simulink model "control_mimo_simulink"  (R2019b)
settings: Solver=ode45  StartTime=0.0  StopTime=60  MaxStep=0.001  RelTol=1e-3
values from neighbouring files (symbols this model uses):
  A = jacobian(F,X)    [codigo_pto_equilibrio_no_lineal.m]
  AL = sys.a    [codigo_pto_equilibrio_no_lineal.m]
  B = jacobian(F,U)    [codigo_pto_equilibrio_no_lineal.m]
  BL = double(Bp)    [codigo_pto_equilibrio_no_lineal.m]
  CL = [2 1 0 ... (first row only)    [codigo_pto_equilibrio_no_lineal.m]
  DL = [0 0 0 ... (first row only)    [codigo_pto_equilibrio_no_lineal.m]
  Kest = Grand*inv(X)    [codigo_pto_equilibrio_no_lineal.m]
  u10 = 1    [codigo_pto_equilibrio_no_lineal.m]
  u20 = 2    [codigo_pto_equilibrio_no_lineal.m]
  u30 = 3    [codigo_pto_equilibrio_no_lineal.m]
  x10n = sqrt((x20n+u20*u30)/a)    [codigo_pto_equilibrio_no_lineal.m]
  x20n = b*x30n - u10*u30    [codigo_pto_equilibrio_no_lineal.m]
  x30n = sqrt((exp(-u10))/c)    [codigo_pto_equilibrio_no_lineal.m]
  xini = [0.2; 0.3; 0.01]    [codigo_pto_equilibrio_no_lineal.m]
undefined symbols (not defined in the file or in its folder): C, D, Kes, Ki
libraries: cstblocks x26
settings Model: Creator=B13  LastModifiedBy=KEVIN ALEJANDRO

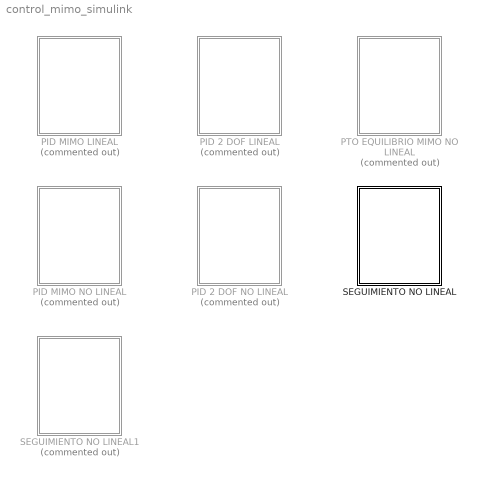
== system control_mimo_simulink ==
  PID 2 DOF LINEAL : Subsystem  Commented=on
  PID 2 DOF NO LINEAL : Subsystem  Commented=on
  PID MIMO LINEAL : Subsystem  Commented=on
  PID MIMO NO LINEAL : Subsystem  Commented=on
  PTO EQUILIBRIO MIMO NO LINEAL : Subsystem  Commented=on
  SEGUIMIENTO NO LINEAL : Subsystem
  SEGUIMIENTO NO LINEAL1 : Subsystem  Commented=on

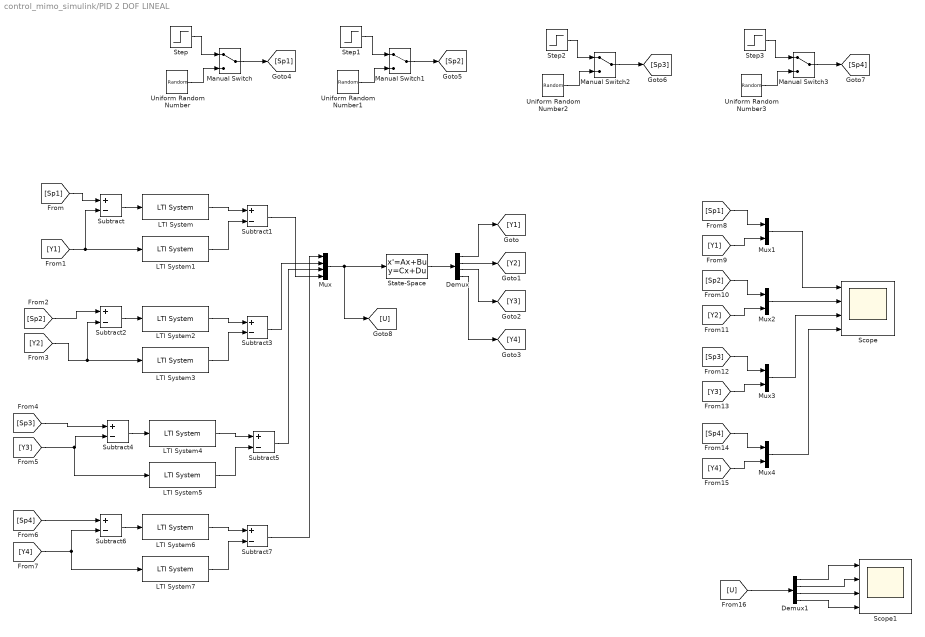
== system control_mimo_simulink/PID 2 DOF LINEAL ==
  Demux : Demux
  Demux1 : Demux
  LTI System : cstblocks/LTI System  sys=C14a  IC=[]
  LTI System1 : cstblocks/LTI System  sys=C14b  IC=[]
  LTI System2 : cstblocks/LTI System  sys=C22a  IC=[]
  LTI System3 : cstblocks/LTI System  sys=C22b  IC=[]
  LTI System4 : cstblocks/LTI System  sys=C33a  IC=[]
  LTI System5 : cstblocks/LTI System  sys=C33b  IC=[]
  LTI System6 : cstblocks/LTI System  sys=C41a  IC=[]
  LTI System7 : cstblocks/LTI System  sys=C41b  IC=[]
  Manual Switch{,1..3} (4 alike) : ManualSwitch
  Mux : Mux
  Mux{1..4} (4 alike) : Mux  Inputs=2
  Scope : Scope  NumInputPorts=4
  Scope1 : Scope  NumInputPorts=4
  State-Space : StateSpace  A=A  B=B  C=C  D=D  InitialCondition=xini
  Step{,1..3} (4 alike) : Step  Time=0  After=0  SampleTime=0
  Subtract{,1..7} (8 alike) : Sum  Inputs=+-
  Uniform Random Number : UniformRandomNumber  SampleTime=500
  Uniform Random Number1 : UniformRandomNumber  SampleTime=700
  Uniform Random Number2 : UniformRandomNumber  SampleTime=900
  Uniform Random Number3 : UniformRandomNumber  SampleTime=1100
  wires:
  Mux2/1 -> Scope/2
  Step1/1 -> Manual Switch1/1
  Manual Switch/1 -> [Sp1]
  [U] -> Demux1/1
  Step2/1 -> Manual Switch2/1
  [Sp2] -> Mux2/1
  Uniform Random Number/1 -> Manual Switch/2
  [Y3] -> Mux3/2
  Demux/4 -> [Y4]
  Mux/1 -> [U], State-Space/1
  Step3/1 -> Manual Switch3/1
  Manual Switch2/1 -> [Sp3]
  Manual Switch1/1 -> [Sp2]
  Manual Switch3/1 -> [Sp4]
  Mux3/1 -> Scope/3
  Uniform Random Number2/1 -> Manual Switch2/2
  Uniform Random Number3/1 -> Manual Switch3/2
  Uniform Random Number1/1 -> Manual Switch1/2
  Step/1 -> Manual Switch/1
  Demux/2 -> [Y2]
  [Y4] -> Mux4/2
  [Sp1] -> Mux1/1
  [Sp4] -> Mux4/1
  Demux/3 -> [Y3]
  State-Space/1 -> Demux/1
  Demux/1 -> [Y1]
  Demux1/3 -> Scope1/3
  Demux1/1 -> Scope1/1
  Demux1/4 -> Scope1/4
  [Sp3] -> Mux3/1
  [Y1] -> Mux1/2
  Mux1/1 -> Scope/1
  Mux4/1 -> Scope/4
  [Y2] -> Mux2/2
  Demux1/2 -> Scope1/2
  [Sp1] -> Subtract/1
  [Y1] -> Subtract/2, LTI System1/1
  Subtract/1 -> LTI System/1
  LTI System/1 -> Subtract1/1
  LTI System1/1 -> Subtract1/2
  Subtract1/1 -> Mux/4
  [Y2] -> Subtract2/2, LTI System3/1
  [Sp2] -> Subtract2/1
  LTI System3/1 -> Subtract3/2
  LTI System2/1 -> Subtract3/1
  Subtract2/1 -> LTI System2/1
  Subtract3/1 -> Mux/2
  [Sp3] -> Subtract4/1
  LTI System5/1 -> Subtract5/2
  LTI System4/1 -> Subtract5/1
  Subtract4/1 -> LTI System4/1
  [Y3] -> LTI System5/1, Subtract4/2
  Subtract5/1 -> Mux/3
  [Sp4] -> Subtract6/1
  LTI System7/1 -> Subtract7/2
  LTI System6/1 -> Subtract7/1
  Subtract6/1 -> LTI System6/1
  [Y4] -> Subtract6/2, LTI System7/1
  Subtract7/1 -> Mux/1

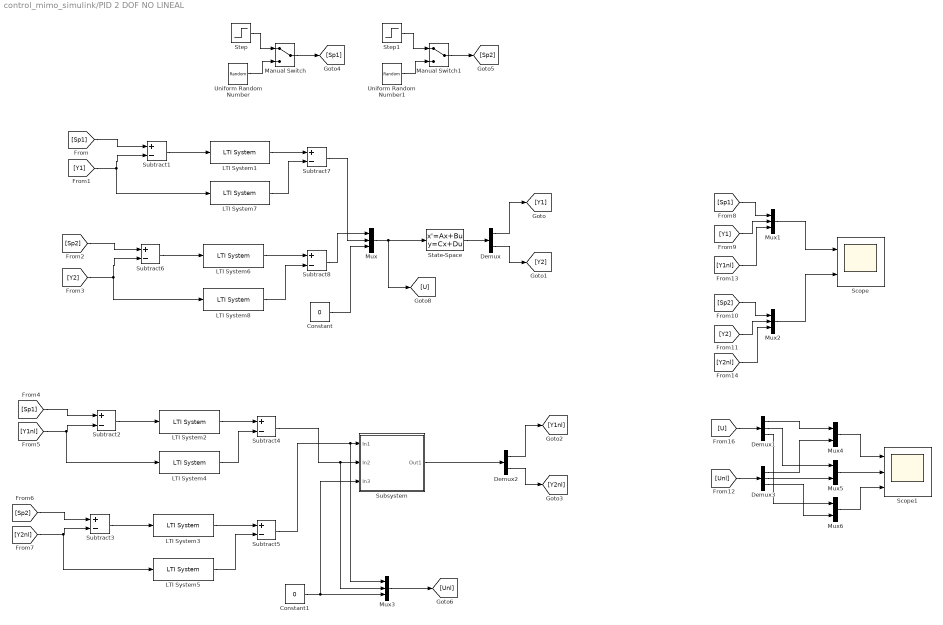
== system control_mimo_simulink/PID 2 DOF NO LINEAL ==
  Constant : Constant  Value=0
  Constant1 : Constant  Value=0
  Demux : Demux  Outputs=2
  Demux1 : Demux  Outputs=3
  Demux2 : Demux  Outputs=2
  Demux3 : Demux  Outputs=3
  LTI System1 : cstblocks/LTI System  sys=C12a  IC=[]
  LTI System2 : cstblocks/LTI System  sys=C12a  IC=[]
  LTI System3 : cstblocks/LTI System  sys=C21a  IC=[]
  LTI System4 : cstblocks/LTI System  sys=C12b  IC=[]
  LTI System5 : cstblocks/LTI System  sys=C21b  IC=[]
  LTI System6 : cstblocks/LTI System  sys=C21a  IC=[]
  LTI System7 : cstblocks/LTI System  sys=C12b  IC=[]
  LTI System8 : cstblocks/LTI System  sys=C21b  IC=[]
  Manual Switch : ManualSwitch
  Manual Switch1 : ManualSwitch
  Mux{,1..3} (4 alike) : Mux  Inputs=3
  Mux4 : Mux  Inputs=2
  Mux5 : Mux  Inputs=2
  Mux6 : Mux  Inputs=2
  Scope : Scope  NumInputPorts=2
  Scope1 : Scope  NumInputPorts=3
  State-Space : StateSpace  A=AL  B=BL  C=CL  D=DL  InitialCondition=xini
  Step : Step  Time=0  After=0  SampleTime=0
  Step1 : Step  Time=0  After=0  SampleTime=0
  Subsystem : Subsystem
  Subtract{1..8} (8 alike) : Sum  Inputs=+-
  Uniform Random Number : UniformRandomNumber  Minimum=-10  Maximum=10  SampleTime=5
  Uniform Random Number1 : UniformRandomNumber  Minimum=-10  Maximum=10  SampleTime=8
  wires:
  Mux2/1 -> Scope/2
  Step1/1 -> Manual Switch1/1
  Manual Switch/1 -> [Sp1]
  [U] -> Demux1/1
  [Sp2] -> Mux2/1
  Uniform Random Number/1 -> Manual Switch/2
  Mux/1 -> [U], State-Space/1
  Manual Switch1/1 -> [Sp2]
  Uniform Random Number1/1 -> Manual Switch1/2
  Step/1 -> Manual Switch/1
  Demux/2 -> [Y2]
  [Sp1] -> Mux1/1
  State-Space/1 -> Demux/1
  Demux/1 -> [Y1]
  [Y1] -> Mux1/2
  Mux1/1 -> Scope/1
  [Y2] -> Mux2/2
  Constant/1 -> Mux/3
  Subtract3/1 -> LTI System3/1
  Demux2/2 -> [Y2nl]
  [Sp1] -> Subtract2/1
  [Y1nl] -> LTI System4/1, Subtract2/2
  Subtract2/1 -> LTI System2/1
  [Sp2] -> Subtract3/1
  Subsystem/1(Out1) -> Demux2/1
  Demux2/1 -> [Y1nl]
  Mux3/1 -> [Unl]
  [Y2nl] -> LTI System5/1, Subtract3/2
  Constant1/1 -> Subsystem/3(In3), Mux3/3
  [Unl] -> Demux3/1
  Demux1/1 -> Mux4/1
  Demux3/1 -> Mux4/2
  Demux1/2 -> Mux5/1
  Demux3/2 -> Mux5/2
  Demux1/3 -> Mux6/1
  Demux3/3 -> Mux6/2
  Mux5/1 -> Scope1/2
  Mux4/1 -> Scope1/1
  Mux6/1 -> Scope1/3
  [Y1nl] -> Mux1/3
  [Y2nl] -> Mux2/3
  LTI System2/1 -> Subtract4/1
  LTI System4/1 -> Subtract4/2
  Subtract4/1 -> Mux3/2, Subsystem/2(In2)
  LTI System3/1 -> Subtract5/1
  LTI System5/1 -> Subtract5/2
  Subtract5/1 -> Mux3/1, Subsystem/1(In1)
  [Y1] -> Subtract1/2, LTI System7/1
  LTI System7/1 -> Subtract7/2
  LTI System8/1 -> Subtract8/2
  Subtract6/1 -> LTI System6/1
  [Sp2] -> Subtract6/1
  LTI System1/1 -> Subtract7/1
  [Sp1] -> Subtract1/1
  LTI System6/1 -> Subtract8/1
  [Y2] -> Subtract6/2, LTI System8/1
  Subtract1/1 -> LTI System1/1
  Subtract7/1 -> Mux/2
  Subtract8/1 -> Mux/1

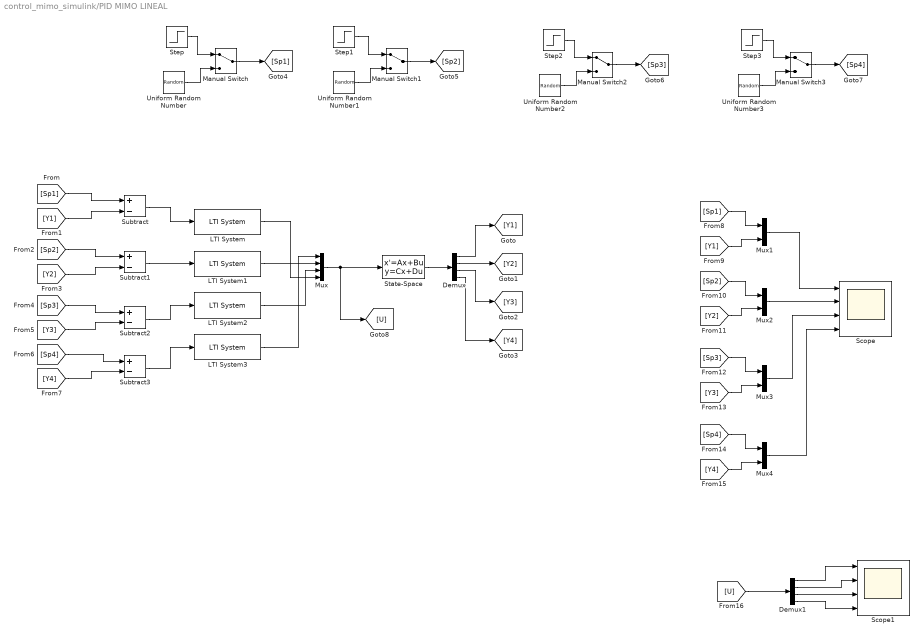
== system control_mimo_simulink/PID MIMO LINEAL ==
  Demux : Demux
  Demux1 : Demux
  LTI System : cstblocks/LTI System  sys=C14  IC=[]
  LTI System1 : cstblocks/LTI System  sys=C22  IC=[]
  LTI System2 : cstblocks/LTI System  sys=C33  IC=[]
  LTI System3 : cstblocks/LTI System  sys=C41  IC=[]
  Manual Switch{,1..3} (4 alike) : ManualSwitch
  Mux : Mux
  Mux{1..4} (4 alike) : Mux  Inputs=2
  Scope : Scope  NumInputPorts=4
  Scope1 : Scope  NumInputPorts=4
  State-Space : StateSpace  A=A  B=B  C=C  D=D  InitialCondition=xini
  Step{,1..3} (4 alike) : Step  Time=0  After=0  SampleTime=0
  Subtract{,1..3} (4 alike) : Sum  Inputs=+-
  Uniform Random Number : UniformRandomNumber  SampleTime=500
  Uniform Random Number1 : UniformRandomNumber  SampleTime=700
  Uniform Random Number2 : UniformRandomNumber  SampleTime=900
  Uniform Random Number3 : UniformRandomNumber  SampleTime=1100
  wires:
  Mux2/1 -> Scope/2
  Step1/1 -> Manual Switch1/1
  Manual Switch/1 -> [Sp1]
  [Y1] -> Subtract/2
  [U] -> Demux1/1
  LTI System/1 -> Mux/4
  Step2/1 -> Manual Switch2/1
  [Sp2] -> Mux2/1
  Uniform Random Number/1 -> Manual Switch/2
  [Y3] -> Mux3/2
  Demux/4 -> [Y4]
  Mux/1 -> [U], State-Space/1
  Step3/1 -> Manual Switch3/1
  Subtract2/1 -> LTI System2/1
  LTI System1/1 -> Mux/2
  Manual Switch2/1 -> [Sp3]
  Manual Switch1/1 -> [Sp2]
  Subtract3/1 -> LTI System3/1
  Manual Switch3/1 -> [Sp4]
  Mux3/1 -> Scope/3
  Subtract1/1 -> LTI System1/1
  Uniform Random Number2/1 -> Manual Switch2/2
  Uniform Random Number3/1 -> Manual Switch3/2
  Uniform Random Number1/1 -> Manual Switch1/2
  Step/1 -> Manual Switch/1
  [Y3] -> Subtract2/2
  [Sp1] -> Subtract/1
  Demux/2 -> [Y2]
  [Y4] -> Mux4/2
  [Sp1] -> Mux1/1
  LTI System2/1 -> Mux/3
  [Sp4] -> Mux4/1
  [Y2] -> Subtract1/2
  [Sp2] -> Subtract1/1
  Demux/3 -> [Y3]
  [Sp3] -> Subtract2/1
  Subtract/1 -> LTI System/1
  [Sp4] -> Subtract3/1
  State-Space/1 -> Demux/1
  LTI System3/1 -> Mux/1
  [Y4] -> Subtract3/2
  Demux/1 -> [Y1]
  Demux1/3 -> Scope1/3
  Demux1/1 -> Scope1/1
  Demux1/4 -> Scope1/4
  [Sp3] -> Mux3/1
  [Y1] -> Mux1/2
  Mux1/1 -> Scope/1
  Mux4/1 -> Scope/4
  [Y2] -> Mux2/2
  Demux1/2 -> Scope1/2

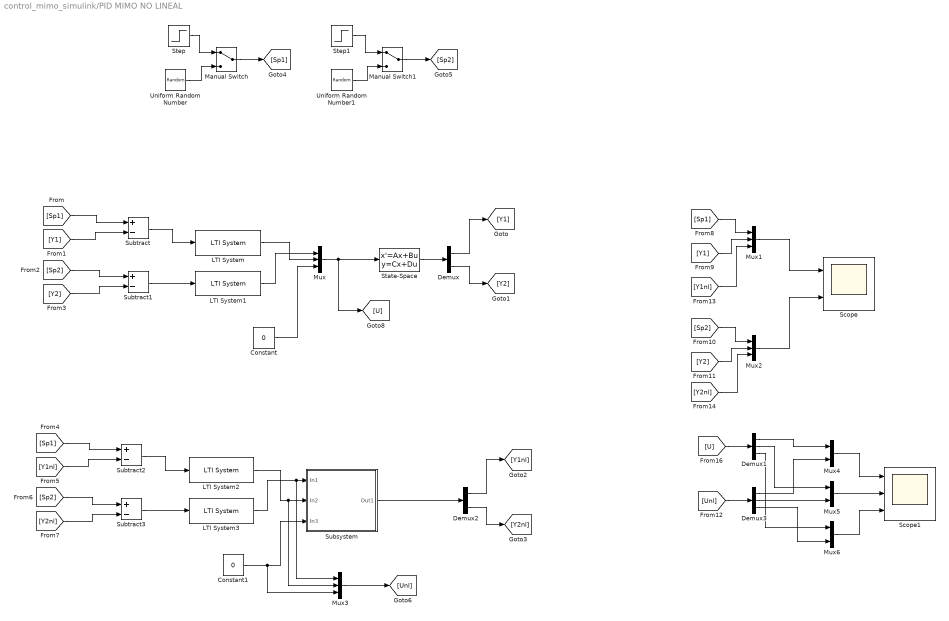
== system control_mimo_simulink/PID MIMO NO LINEAL ==
  Constant : Constant  Value=0
  Constant1 : Constant  Value=0
  Demux : Demux  Outputs=2
  Demux1 : Demux  Outputs=3
  Demux2 : Demux  Outputs=2
  Demux3 : Demux  Outputs=3
  LTI System : cstblocks/LTI System  sys=C12  IC=[]
  LTI System1 : cstblocks/LTI System  sys=C21  IC=[]
  LTI System2 : cstblocks/LTI System  sys=C12  IC=[]
  LTI System3 : cstblocks/LTI System  sys=C21  IC=[]
  Manual Switch : ManualSwitch
  Manual Switch1 : ManualSwitch
  Mux{,1..3} (4 alike) : Mux  Inputs=3
  Mux4 : Mux  Inputs=2
  Mux5 : Mux  Inputs=2
  Mux6 : Mux  Inputs=2
  Scope : Scope  NumInputPorts=2
  Scope1 : Scope  NumInputPorts=3
  State-Space : StateSpace  A=AL  B=BL  C=CL  D=DL  InitialCondition=xini
  Step : Step  Time=0  After=0  SampleTime=0
  Step1 : Step  Time=0  After=0  SampleTime=0
  Subsystem : Subsystem
  Subtract{,1..3} (4 alike) : Sum  Inputs=+-
  Uniform Random Number : UniformRandomNumber  Minimum=-2  Maximum=2  SampleTime=5
  Uniform Random Number1 : UniformRandomNumber  Minimum=-2  Maximum=2  SampleTime=8
  wires:
  Mux2/1 -> Scope/2
  Step1/1 -> Manual Switch1/1
  Manual Switch/1 -> [Sp1]
  [Y1] -> Subtract/2
  [U] -> Demux1/1
  [Sp2] -> Mux2/1
  Uniform Random Number/1 -> Manual Switch/2
  Mux/1 -> [U], State-Space/1
  Manual Switch1/1 -> [Sp2]
  Subtract1/1 -> LTI System1/1
  Uniform Random Number1/1 -> Manual Switch1/2
  Step/1 -> Manual Switch/1
  [Sp1] -> Subtract/1
  Demux/2 -> [Y2]
  [Sp1] -> Mux1/1
  [Y2] -> Subtract1/2
  [Sp2] -> Subtract1/1
  Subtract/1 -> LTI System/1
  State-Space/1 -> Demux/1
  Demux/1 -> [Y1]
  [Y1] -> Mux1/2
  Mux1/1 -> Scope/1
  [Y2] -> Mux2/2
  LTI System/1 -> Mux/2
  LTI System1/1 -> Mux/1
  Constant/1 -> Mux/3
  Subtract3/1 -> LTI System3/1
  Demux2/2 -> [Y2nl]
  [Sp1] -> Subtract2/1
  [Y1nl] -> Subtract2/2
  Subtract2/1 -> LTI System2/1
  [Sp2] -> Subtract3/1
  Subsystem/1(Out1) -> Demux2/1
  Demux2/1 -> [Y1nl]
  Mux3/1 -> [Unl]
  [Y2nl] -> Subtract3/2
  LTI System2/1 -> Mux3/2, Subsystem/2(In2)
  LTI System3/1 -> Mux3/1, Subsystem/1(In1)
  Constant1/1 -> Mux3/3, Subsystem/3(In3)
  [Unl] -> Demux3/1
  Demux1/1 -> Mux4/1
  Demux3/1 -> Mux4/2
  Demux1/2 -> Mux5/1
  Demux3/2 -> Mux5/2
  Demux1/3 -> Mux6/1
  Demux3/3 -> Mux6/2
  Mux5/1 -> Scope1/2
  Mux4/1 -> Scope1/1
  Mux6/1 -> Scope1/3
  [Y1nl] -> Mux1/3
  [Y2nl] -> Mux2/3

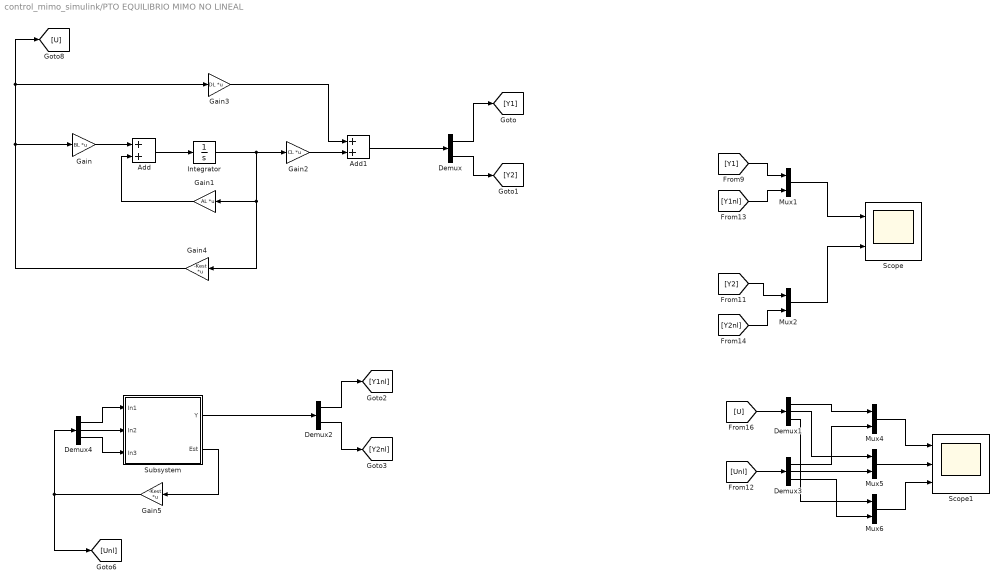
== system control_mimo_simulink/PTO EQUILIBRIO MIMO NO LINEAL ==
  Add : Sum
  Add1 : Sum
  Demux : Demux  Outputs=2
  Demux1 : Demux  Outputs=3
  Demux2 : Demux  Outputs=2
  Demux3 : Demux  Outputs=3
  Demux4 : Demux  Outputs=3
  Gain : Gain  Gain=BL  Multiplication=Matrix(K*u)
  Gain1 : Gain  Gain=AL  Multiplication=Matrix(K*u)
  Gain2 : Gain  Gain=CL  Multiplication=Matrix(K*u)
  Gain3 : Gain  Gain=DL  Multiplication=Matrix(K*u)
  Gain4 : Gain  Gain=-Kest  Multiplication=Matrix(K*u)
  Gain5 : Gain  Gain=-Kest  Multiplication=Matrix(K*u)
  Integrator : Integrator  InitialCondition=xini
  Mux{1..2,4..6} (5 alike) : Mux  Inputs=2
  Scope : Scope  NumInputPorts=2
  Scope1 : Scope  NumInputPorts=3
  Subsystem : Subsystem
  wires:
  Mux2/1 -> Scope/2
  [U] -> Demux1/1
  Demux/2 -> [Y2]
  Add1/1 -> Demux/1
  Demux/1 -> [Y1]
  Mux1/1 -> Scope/1
  Demux2/2 -> [Y2nl]
  Subsystem/1(Y) -> Demux2/1
  Demux2/1 -> [Y1nl]
  [Unl] -> Demux3/1
  Demux1/1 -> Mux4/1
  Demux3/1 -> Mux4/2
  Demux1/2 -> Mux5/1
  Demux3/2 -> Mux5/2
  Demux1/3 -> Mux6/1
  Demux3/3 -> Mux6/2
  Mux5/1 -> Scope1/2
  Mux4/1 -> Scope1/1
  Mux6/1 -> Scope1/3
  Gain/1 -> Add/1
  Add/1 -> Integrator/1
  Gain1/1 -> Add/2
  Integrator/1 -> Gain2/1, Gain4/1, Gain1/1
  Gain2/1 -> Add1/2
  Gain3/1 -> Add1/1
  Gain4/1 -> Gain/1, [U], Gain3/1
  Subsystem/2(Est) -> Gain5/1
  Demux4/2 -> Subsystem/2(In2)
  Demux4/1 -> Subsystem/1(In1)
  Demux4/3 -> Subsystem/3(In3)
  Gain5/1 -> Demux4/1, [Unl]
  [Y1] -> Mux1/1
  [Y1nl] -> Mux1/2
  [Y2] -> Mux2/1
  [Y2nl] -> Mux2/2

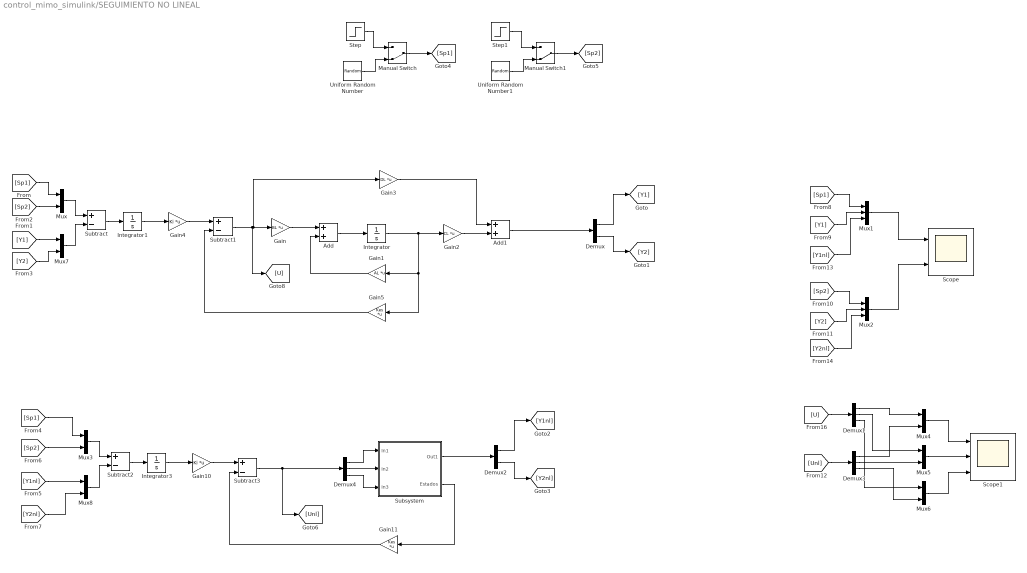
== system control_mimo_simulink/SEGUIMIENTO NO LINEAL ==
  Add : Sum
  Add1 : Sum
  Demux : Demux  Outputs=2
  Demux1 : Demux  Outputs=3
  Demux2 : Demux  Outputs=2
  Demux3 : Demux  Outputs=3
  Demux4 : Demux  Outputs=3
  Gain : Gain  Gain=BL  Multiplication=Matrix(K*u)
  Gain1 : Gain  Gain=AL  Multiplication=Matrix(K*u)
  Gain10 : Gain  Gain=Ki  Multiplication=Matrix(K*u)
  Gain11 : Gain  Gain=Kes  Multiplication=Matrix(K*u)
  Gain2 : Gain  Gain=CL  Multiplication=Matrix(K*u)
  Gain3 : Gain  Gain=DL  Multiplication=Matrix(K*u)
  Gain4 : Gain  Gain=Ki  Multiplication=Matrix(K*u)
  Gain5 : Gain  Gain=Kes  Multiplication=Matrix(K*u)
  Integrator : Integrator
  Integrator1 : Integrator
  Integrator3 : Integrator
  Manual Switch : ManualSwitch  CurrentSetting=0
  Manual Switch1 : ManualSwitch  CurrentSetting=0
  Mux{,3..8} (7 alike) : Mux  Inputs=2
  Mux1 : Mux  Inputs=3
  Mux2 : Mux  Inputs=3
  Scope : Scope  NumInputPorts=2
  Scope1 : Scope  NumInputPorts=3
  Step : Step  Time=0  SampleTime=0
  Step1 : Step  Time=0  SampleTime=0
  Subsystem : Subsystem
  Subtract{,1..3} (4 alike) : Sum  Inputs=+-
  Uniform Random Number : UniformRandomNumber  Minimum=-5  Maximum=5  SampleTime=5
  Uniform Random Number1 : UniformRandomNumber  Minimum=-5  Maximum=5  SampleTime=8
  wires:
  Mux2/1 -> Scope/2
  Step1/1 -> Manual Switch1/1
  Manual Switch/1 -> [Sp1]
  [U] -> Demux1/1
  [Sp2] -> Mux2/1
  Uniform Random Number/1 -> Manual Switch/2
  Manual Switch1/1 -> [Sp2]
  Uniform Random Number1/1 -> Manual Switch1/2
  Step/1 -> Manual Switch/1
  Demux/2 -> [Y2]
  [Sp1] -> Mux1/1
  Add1/1 -> Demux/1
  Demux/1 -> [Y1]
  [Y1] -> Mux1/2
  Mux1/1 -> Scope/1
  [Y2] -> Mux2/2
  Demux2/2 -> [Y2nl]
  Subsystem/1(Out1) -> Demux2/1
  Demux2/1 -> [Y1nl]
  [Unl] -> Demux3/1
  Demux1/1 -> Mux4/1
  Demux3/1 -> Mux4/2
  Demux1/2 -> Mux5/1
  Demux3/2 -> Mux5/2
  Demux1/3 -> Mux6/1
  Demux3/3 -> Mux6/2
  Mux5/1 -> Scope1/2
  Mux4/1 -> Scope1/1
  Mux6/1 -> Scope1/3
  [Y1nl] -> Mux1/3
  [Y2nl] -> Mux2/3
  Add/1 -> Integrator/1
  Integrator/1 -> Gain2/1, Gain5/1, Gain1/1
  Gain/1 -> Add/1
  Gain2/1 -> Add1/2
  Gain1/1 -> Add/2
  Gain3/1 -> Add1/1
  [Sp1] -> Mux/1
  [Sp2] -> Mux/2
  Mux/1 -> Subtract/1
  [Y1] -> Mux7/1
  [Y2] -> Mux7/2
  Mux7/1 -> Subtract/2
  Subtract/1 -> Integrator1/1
  Integrator1/1 -> Gain4/1
  Gain4/1 -> Subtract1/1
  Subtract1/1 -> [U], Gain3/1, Gain/1
  Gain5/1 -> Subtract1/2
  Mux3/1 -> Subtract2/1
  Subtract3/1 -> [Unl], Demux4/1
  Integrator3/1 -> Gain10/1
  Gain10/1 -> Subtract3/1
  [Y1nl] -> Mux8/1
  Subtract2/1 -> Integrator3/1
  [Sp2] -> Mux3/2
  [Y2nl] -> Mux8/2
  Mux8/1 -> Subtract2/2
  Gain11/1 -> Subtract3/2
  [Sp1] -> Mux3/1
  Demux4/1 -> Subsystem/1(In1)
  Demux4/2 -> Subsystem/2(In2)
  Demux4/3 -> Subsystem/3(In3)
  Subsystem/2(Estados) -> Gain11/1

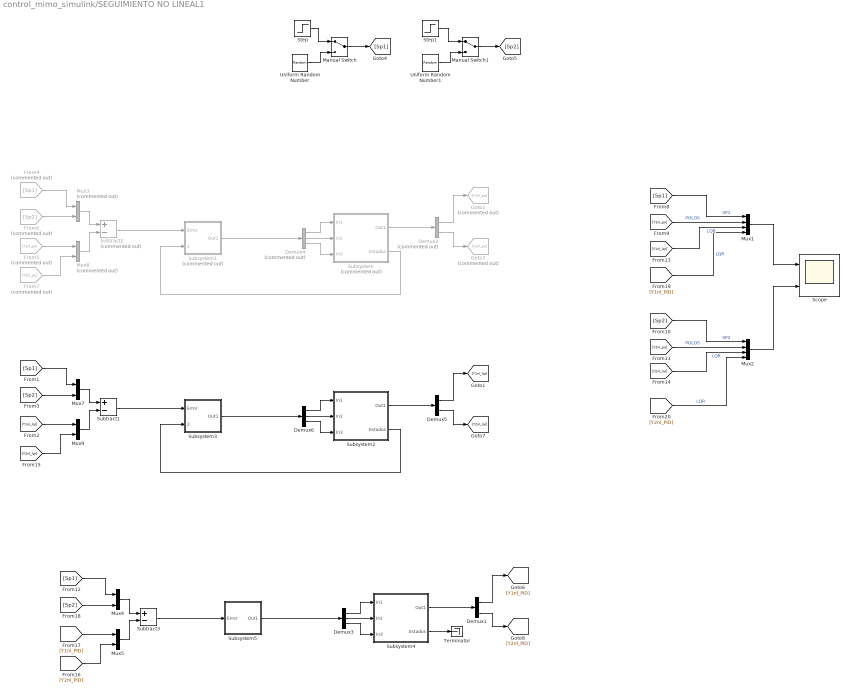
== system control_mimo_simulink/SEGUIMIENTO NO LINEAL1 ==
  Demux1 : Demux  Outputs=2
  Demux2 : Demux  Commented=on  Outputs=2
  Demux3 : Demux  Outputs=3
  Demux4 : Demux  Commented=on  Outputs=3
  Demux5 : Demux  Outputs=2
  Demux6 : Demux  Outputs=3
  From4 : From  Commented=on  GotoTag=Sp1
  From5 : From  Commented=on  GotoTag=Y1nl_po
  From6 : From  Commented=on  GotoTag=Sp2
  From7 : From  Commented=on  GotoTag=Y2nl_po
  Goto2 : Goto  Commented=on  GotoTag=Y1nl_po
  Goto3 : Goto  Commented=on  GotoTag=Y2nl_po
  Manual Switch : ManualSwitch
  Manual Switch1 : ManualSwitch
  Mux1 : Mux
  Mux2 : Mux
  Mux3 : Mux  Commented=on  Inputs=2
  Mux{4..5,7,9} (4 alike) : Mux  Inputs=2
  Mux8 : Mux  Commented=on  Inputs=2
  Scope : Scope  NumInputPorts=2
  Step : Step  Time=0  After=0  SampleTime=0
  Step1 : Step  Time=0  After=0  SampleTime=0
  Subsystem : Subsystem  Commented=on  mask{xini=[-0.2; 0.4; 0.5]}
      mask prompts: xini "Condiciones Iniciales"
      mask init:
      | a = 1;
      | b = 1;
      | c = 1;
      | u10 = 1;
      | u20 = 2;
      | u30 = 3;
      | x30n = sqrt(exp(-u10)/c);
      | x20n = b*x30n - u10*u30;
      | x10n = sqrt((x20n+u20*u30)/a);
      | 
      | CL = [2 1 0;
      |       0 2 4];
      | DL = zeros(2,3);
  Subsystem1 : Subsystem  Commented=on  mask(Controlador Por ubicación de polos){Ki=[-0.0989933962140377,-8.06282500675100;12.4995779729889,-12.9300009318227;-1.38348094674764,13.2646252136592], Kes=[0.130559475600719,-6.41283506023148,-13.5686995839442;5.34408621711497,-2.83651918164370,-25.5201366498674;-0.745661452356591,8.78232145962737,21.1522453168287]}
      mask prompts: Ki "Ganancia Integral"; Kes "Ganancia Estados"
  Subsystem2 : Subsystem  mask{xini=[-0.2; 0.4; 0.5]}
      mask prompts: xini "Condiciones Iniciales"
      mask init:
      | a = 1;
      | b = 1;
      | c = 1;
      | u10 = 1;
      | u20 = 2;
      | u30 = 3;
      | x30n = sqrt(exp(-u10)/c);
      | x20n = b*x30n - u10*u30;
      | x10n = sqrt((x20n+u20*u30)/a);
      | 
      | CL = [2 1 0;
      |       0 2 4];
      | DL = zeros(2,3);
  Subsystem3 : Subsystem  mask(Controlador Por LQR){Ki=[-0.924625421721551,-2.97969985505990;2.73014662919296,-0.590365331044532;1.30052574469426,-0.879123170924667], Kes=[-0.297327653520697,-3.06798399298749,-5.64896908720005;1.14760514998956,0.574650427752299,-2.26152437343483;0.573519957408942,-0.963537616124815,1.13429595603273]}
      mask prompts: Ki "Ganancia Integral"; Kes "Ganancia Estados"
  Subsystem4 : Subsystem  mask{xini=[-0.2; 0.4; 0.5]}
      mask prompts: xini "Condiciones Iniciales"
      mask init:
      | a = 1;
      | b = 1;
      | c = 1;
      | u10 = 1;
      | u20 = 2;
      | u30 = 3;
      | x30n = sqrt(exp(-u10)/c);
      | x20n = b*x30n - u10*u30;
      | x10n = sqrt((x20n+u20*u30)/a);
      | 
      | CL = [2 1 0;
      |       0 2 4];
      | DL = zeros(2,3);
  Subsystem5 : Subsystem  mask(Controlador Por PID){C12=tf([0.17,0.986],[1 0]), C21=tf([-0.34,-0.986],[1,0])}
      mask prompts: C12 "Controlador 1"; C21 "Controlador 2"
  Subtract1 : Sum  Inputs=+-
  Subtract2 : Sum  Commented=on  Inputs=+-
  Subtract3 : Sum  Inputs=+-
  Terminator : Terminator
  Uniform Random Number : UniformRandomNumber  SampleTime=5
  Uniform Random Number1 : UniformRandomNumber  SampleTime=8
  wires:
  Mux2/1 -> Scope/2
  Step1/1 -> Manual Switch1/1
  Manual Switch/1 -> [Sp1]
  [Sp2] -> Mux2/1  "SP2"
  Uniform Random Number/1 -> Manual Switch/2
  Manual Switch1/1 -> [Sp2]
  Uniform Random Number1/1 -> Manual Switch1/2
  Step/1 -> Manual Switch/1
  [Sp1] -> Mux1/1  "SP1"
  [Y1nl_po] -> Mux1/2  "POLOS"
  Mux1/1 -> Scope/1
  [Y2nl_po] -> Mux2/2  "POLOS"
  Demux2/2 -> Goto3/1
  Subsystem/1(Out1) -> Demux2/1
  Demux2/1 -> Goto2/1
  [Y1nl_lqr] -> Mux1/3  "LQR"
  [Y2nl_lqr] -> Mux2/3  "LQR"
  Mux3/1 -> Subtract2/1
  From5/1 -> Mux8/1
  From6/1 -> Mux3/2
  From7/1 -> Mux8/2
  Mux8/1 -> Subtract2/2
  From4/1 -> Mux3/1
  Demux4/1 -> Subsystem/1(In1)
  Demux4/2 -> Subsystem/2(In2)
  Demux4/3 -> Subsystem/3(In3)
  Subtract2/1 -> Subsystem1/1(Error)
  Subsystem1/1(Out1) -> Demux4/1
  Subsystem/2(Estados) -> Subsystem1/2(Estados)
  Demux6/3 -> Subsystem2/3(In3)
  [Y1nl_lqr] -> Mux9/1
  [Y2nl_lqr] -> Mux9/2
  Demux6/2 -> Subsystem2/2(In2)
  Demux6/1 -> Subsystem2/1(In1)
  Demux5/2 -> [Y2nl_lqr]
  Mux9/1 -> Subtract1/2
  Mux7/1 -> Subtract1/1
  Subsystem2/1(Out1) -> Demux5/1
  Subtract1/1 -> Subsystem3/1(Error)
  Demux5/1 -> [Y1nl_lqr]
  Subsystem3/1(Out1) -> Demux6/1
  [Sp2] -> Mux7/2
  [Sp1] -> Mux7/1
  Subsystem2/2(Estados) -> Subsystem3/2(Estados)
  [Sp2] -> Mux4/2
  Demux1/1 -> [Y1nl_PID]
  [Sp1] -> Mux4/1
  Subsystem4/1(Out1) -> Demux1/1
  Mux5/1 -> Subtract3/2
  Mux4/1 -> Subtract3/1
  [Y2nl_PID] -> Mux5/2
  Subtract3/1 -> Subsystem5/1(Error)
  [Y1nl_PID] -> Mux5/1
  Demux1/2 -> [Y2nl_PID]
  Demux3/1 -> Subsystem4/1(In1)
  Demux3/2 -> Subsystem4/2(In2)
  Demux3/3 -> Subsystem4/3(In3)
  Subsystem4/2(Estados) -> Terminator/1
  Subsystem5/1(Out1) -> Demux3/1
  [Y1nl_PID] -> Mux1/4  "LQR"
  [Y2nl_PID] -> Mux2/4  "LQR"

== system control_mimo_simulink/PID 2 DOF NO LINEAL/Subsystem ==
  In1 : Inport
  In2 : Inport  Port=2
  In3 : Inport  Port=3
  Add : Sum
  Add1 : Sum
  Add2 : Sum
  Constant : Constant  Value=[x10n; x20n; x30n]
  Constant1 : Constant  Value=u10
  Constant2 : Constant  Value=u20
  Constant3 : Constant  Value=u30
  Gain : Gain  Gain=CL  Multiplication=Matrix(K*u)
  Integrator : Integrator  InitialCondition=[x10n; x20n; x30n]+xini
  MATLAB Function : MATLAB Function  TreatAsAtomicUnit=on
  Mux : Mux  Inputs=3
  Subtract : Sum  Inputs=+-
  Out1 : Outport
  wires:
  Integrator/1 -> MATLAB Function/1(x), Subtract/1
  Constant/1 -> Subtract/2
  Subtract/1 -> Gain/1
  Gain/1 -> Out1/1
  MATLAB Function/1(F) -> Integrator/1
  Add/1 -> Mux/1
  In1/1 -> Add/2
  Constant1/1 -> Add/1
  Constant2/1 -> Add1/1
  In2/1 -> Add1/2
  Add1/1 -> Mux/2
  Constant3/1 -> Add2/1
  In3/1 -> Add2/2
  Add2/1 -> Mux/3
  Mux/1 -> MATLAB Function/2(u)

== system control_mimo_simulink/PID MIMO NO LINEAL/Subsystem ==
  In1 : Inport
  In2 : Inport  Port=2
  In3 : Inport  Port=3
  Add : Sum
  Add1 : Sum
  Add2 : Sum
  Constant : Constant  Value=[x10n; x20n; x30n]
  Constant1 : Constant  Value=u10
  Constant2 : Constant  Value=u20
  Constant3 : Constant  Value=u30
  Gain : Gain  Gain=CL  Multiplication=Matrix(K*u)
  Integrator : Integrator  InitialCondition=[x10n; x20n; x30n]+xini
  MATLAB Function : MATLAB Function  TreatAsAtomicUnit=on
  Mux : Mux  Inputs=3
  Subtract : Sum  Inputs=+-
  Out1 : Outport
  wires:
  Integrator/1 -> MATLAB Function/1(x), Subtract/1
  Constant/1 -> Subtract/2
  Subtract/1 -> Gain/1
  Gain/1 -> Out1/1
  MATLAB Function/1(F) -> Integrator/1
  Add/1 -> Mux/1
  In1/1 -> Add/2
  Constant1/1 -> Add/1
  Constant2/1 -> Add1/1
  In2/1 -> Add1/2
  Add1/1 -> Mux/2
  Constant3/1 -> Add2/1
  In3/1 -> Add2/2
  Add2/1 -> Mux/3
  Mux/1 -> MATLAB Function/2(u)

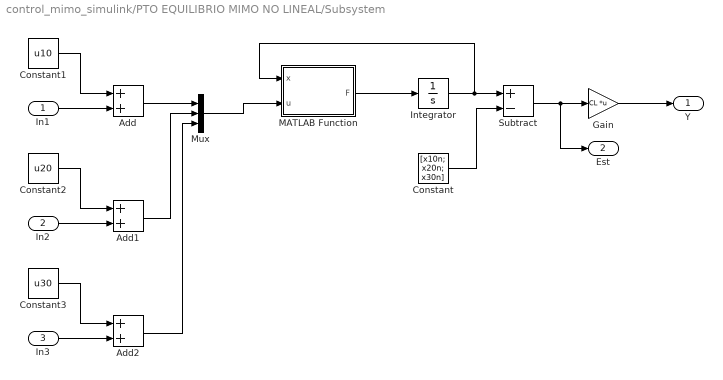
== system control_mimo_simulink/PTO EQUILIBRIO MIMO NO LINEAL/Subsystem ==
  In1 : Inport
  In2 : Inport  Port=2
  In3 : Inport  Port=3
  Add : Sum
  Add1 : Sum
  Add2 : Sum
  Constant : Constant  Value=[x10n; x20n; x30n]
  Constant1 : Constant  Value=u10
  Constant2 : Constant  Value=u20
  Constant3 : Constant  Value=u30
  Gain : Gain  Gain=CL  Multiplication=Matrix(K*u)
  Integrator : Integrator  InitialCondition=[x10n; x20n; x30n]+xini
  MATLAB Function : MATLAB Function  TreatAsAtomicUnit=on
  Mux : Mux  Inputs=3
  Subtract : Sum  Inputs=+-
  Y : Outport
  Est : Outport  Port=2
  wires:
  Integrator/1 -> Subtract/1, MATLAB Function/1(x)
  Constant/1 -> Subtract/2
  Subtract/1 -> Est/1, Gain/1
  Gain/1 -> Y/1
  MATLAB Function/1(F) -> Integrator/1
  Add/1 -> Mux/1
  In1/1 -> Add/2
  Constant1/1 -> Add/1
  Constant2/1 -> Add1/1
  In2/1 -> Add1/2
  Add1/1 -> Mux/2
  Constant3/1 -> Add2/1
  In3/1 -> Add2/2
  Add2/1 -> Mux/3
  Mux/1 -> MATLAB Function/2(u)

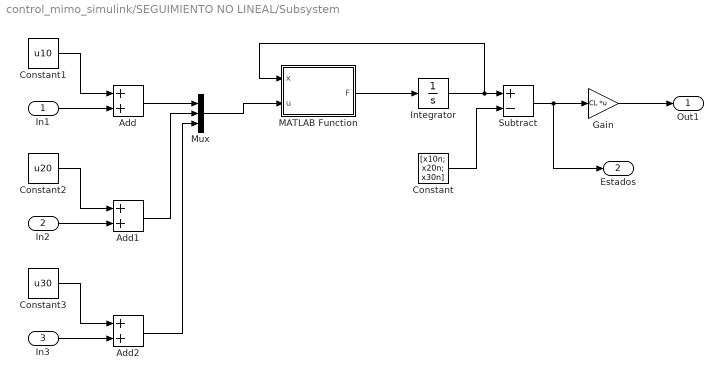
== system control_mimo_simulink/SEGUIMIENTO NO LINEAL/Subsystem ==
  In1 : Inport
  In2 : Inport  Port=2
  In3 : Inport  Port=3
  Add : Sum
  Add1 : Sum
  Add2 : Sum
  Constant : Constant  Value=[x10n; x20n; x30n]
  Constant1 : Constant  Value=u10
  Constant2 : Constant  Value=u20
  Constant3 : Constant  Value=u30
  Gain : Gain  Gain=CL  Multiplication=Matrix(K*u)
  Integrator : Integrator  InitialCondition=[x10n; x20n; x30n]
  MATLAB Function : MATLAB Function  TreatAsAtomicUnit=on
  Mux : Mux  Inputs=3
  Subtract : Sum  Inputs=+-
  Out1 : Outport
  Estados : Outport  Port=2
  wires:
  Integrator/1 -> MATLAB Function/1(x), Subtract/1
  Constant/1 -> Subtract/2
  Subtract/1 -> Estados/1, Gain/1
  Gain/1 -> Out1/1
  MATLAB Function/1(F) -> Integrator/1
  Add/1 -> Mux/1
  In1/1 -> Add/2
  Constant1/1 -> Add/1
  Constant2/1 -> Add1/1
  In2/1 -> Add1/2
  Add1/1 -> Mux/2
  Constant3/1 -> Add2/1
  In3/1 -> Add2/2
  Add2/1 -> Mux/3
  Mux/1 -> MATLAB Function/2(u)

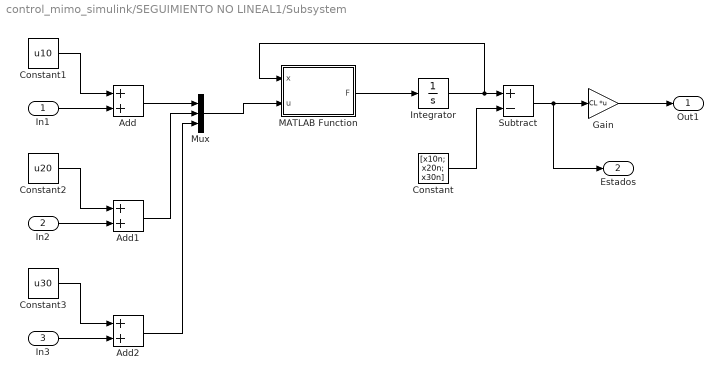
== system control_mimo_simulink/SEGUIMIENTO NO LINEAL1/Subsystem ==
  In1 : Inport
  In2 : Inport  Port=2
  In3 : Inport  Port=3
  Add : Sum
  Add1 : Sum
  Add2 : Sum
  Constant : Constant  Value=[x10n; x20n; x30n]
  Constant1 : Constant  Value=u10
  Constant2 : Constant  Value=u20
  Constant3 : Constant  Value=u30
  Gain : Gain  Gain=CL  Multiplication=Matrix(K*u)
  Integrator : Integrator  InitialCondition=[x10n; x20n; x30n]+xini
  MATLAB Function : MATLAB Function  TreatAsAtomicUnit=on
  Mux : Mux  Inputs=3
  Subtract : Sum  Inputs=+-
  Out1 : Outport
  Estados : Outport  Port=2
  wires:
  Integrator/1 -> MATLAB Function/1(x), Subtract/1
  Constant/1 -> Subtract/2
  Subtract/1 -> Estados/1, Gain/1
  Gain/1 -> Out1/1
  MATLAB Function/1(F) -> Integrator/1
  Add/1 -> Mux/1
  In1/1 -> Add/2
  Constant1/1 -> Add/1
  Constant2/1 -> Add1/1
  In2/1 -> Add1/2
  Add1/1 -> Mux/2
  Constant3/1 -> Add2/1
  In3/1 -> Add2/2
  Add2/1 -> Mux/3
  Mux/1 -> MATLAB Function/2(u)

== system control_mimo_simulink/SEGUIMIENTO NO LINEAL1/Subsystem1 ==
  Error : Inport
  Estados : Inport  Port=2
  Gain10 : Gain  Gain=Ki  Multiplication=Matrix(K*u)
  Gain11 : Gain  Gain=Kes  Multiplication=Matrix(K*u)
  Integrator3 : Integrator
  Subtract3 : Sum  Inputs=+-
  Out1 : Outport
  wires:
  Gain11/1 -> Subtract3/2
  Gain10/1 -> Subtract3/1
  Integrator3/1 -> Gain10/1
  Error/1 -> Integrator3/1
  Subtract3/1 -> Out1/1
  Estados/1 -> Gain11/1

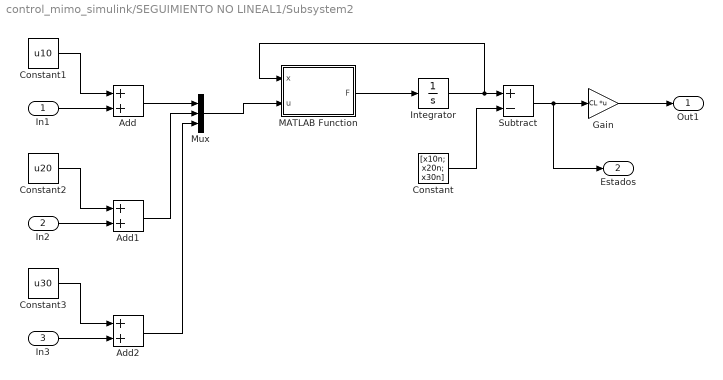
== system control_mimo_simulink/SEGUIMIENTO NO LINEAL1/Subsystem2 ==
  In1 : Inport
  In2 : Inport  Port=2
  In3 : Inport  Port=3
  Add : Sum
  Add1 : Sum
  Add2 : Sum
  Constant : Constant  Value=[x10n; x20n; x30n]
  Constant1 : Constant  Value=u10
  Constant2 : Constant  Value=u20
  Constant3 : Constant  Value=u30
  Gain : Gain  Gain=CL  Multiplication=Matrix(K*u)
  Integrator : Integrator  InitialCondition=[x10n; x20n; x30n]+xini
  MATLAB Function : MATLAB Function  TreatAsAtomicUnit=on
  Mux : Mux  Inputs=3
  Subtract : Sum  Inputs=+-
  Out1 : Outport
  Estados : Outport  Port=2
  wires:
  Integrator/1 -> MATLAB Function/1(x), Subtract/1
  Constant/1 -> Subtract/2
  Subtract/1 -> Estados/1, Gain/1
  Gain/1 -> Out1/1
  MATLAB Function/1(F) -> Integrator/1
  Add/1 -> Mux/1
  In1/1 -> Add/2
  Constant1/1 -> Add/1
  Constant2/1 -> Add1/1
  In2/1 -> Add1/2
  Add1/1 -> Mux/2
  Constant3/1 -> Add2/1
  In3/1 -> Add2/2
  Add2/1 -> Mux/3
  Mux/1 -> MATLAB Function/2(u)

== system control_mimo_simulink/SEGUIMIENTO NO LINEAL1/Subsystem3 ==
  Error : Inport
  Estados : Inport  Port=2
  Gain10 : Gain  Gain=Ki  Multiplication=Matrix(K*u)
  Gain11 : Gain  Gain=Kes  Multiplication=Matrix(K*u)
  Integrator3 : Integrator
  Subtract3 : Sum  Inputs=+-
  Out1 : Outport
  wires:
  Gain11/1 -> Subtract3/2
  Gain10/1 -> Subtract3/1
  Integrator3/1 -> Gain10/1
  Error/1 -> Integrator3/1
  Subtract3/1 -> Out1/1
  Estados/1 -> Gain11/1

== system control_mimo_simulink/SEGUIMIENTO NO LINEAL1/Subsystem4 ==
  In1 : Inport
  In2 : Inport  Port=2
  In3 : Inport  Port=3
  Add : Sum
  Add1 : Sum
  Add2 : Sum
  Constant : Constant  Value=[x10n; x20n; x30n]
  Constant1 : Constant  Value=u10
  Constant2 : Constant  Value=u20
  Constant3 : Constant  Value=u30
  Gain : Gain  Gain=CL  Multiplication=Matrix(K*u)
  Integrator : Integrator  InitialCondition=[x10n; x20n; x30n]+xini
  MATLAB Function : MATLAB Function  TreatAsAtomicUnit=on
  Mux : Mux  Inputs=3
  Subtract : Sum  Inputs=+-
  Out1 : Outport
  Estados : Outport  Port=2
  wires:
  Integrator/1 -> MATLAB Function/1(x), Subtract/1
  Constant/1 -> Subtract/2
  Subtract/1 -> Estados/1, Gain/1
  Gain/1 -> Out1/1
  MATLAB Function/1(F) -> Integrator/1
  Add/1 -> Mux/1
  In1/1 -> Add/2
  Constant1/1 -> Add/1
  Constant2/1 -> Add1/1
  In2/1 -> Add1/2
  Add1/1 -> Mux/2
  Constant3/1 -> Add2/1
  In3/1 -> Add2/2
  Add2/1 -> Mux/3
  Mux/1 -> MATLAB Function/2(u)

== system control_mimo_simulink/SEGUIMIENTO NO LINEAL1/Subsystem5 ==
  Error : Inport
  Constant1 : Constant  Value=0
  Demux : Demux  Outputs=2
  LTI System2 : cstblocks/LTI System  sys=C12  IC=[]
  LTI System3 : cstblocks/LTI System  sys=C21  IC=[]
  Mux : Mux  Inputs=3
  Out1 : Outport
  wires:
  Constant1/1 -> Mux/3
  Demux/1 -> LTI System2/1
  Demux/2 -> LTI System3/1
  Error/1 -> Demux/1
  LTI System2/1 -> Mux/2
  LTI System3/1 -> Mux/1
  Mux/1 -> Out1/1

== matlab function control_mimo_simulink/PID 2 DOF NO LINEAL/Subsystem/MATLAB Function ==
  data: x input; u input; F output
function F = fcn(x,u)
x1 = x(1);
x2 = x(2);
x3 = x(3);
u1 = u(1);
u2 = u(2);
u3 = u(3);
a = 1;
b = 1;
c = 1;
f1 = -a*x1^2 + x2 + u2*u3;
f2 = -x2 + b*x3 - u1*u3;
f3 = -c*x3^2 + exp(-u1);
F = [f1; f2; f3];

== matlab function control_mimo_simulink/PID MIMO NO LINEAL/Subsystem/MATLAB Function ==
  data: x input; u input; F output
function F = fcn(x,u)
x1 = x(1);
x2 = x(2);
x3 = x(3);
u1 = u(1);
u2 = u(2);
u3 = u(3);
a = 1;
b = 1;
c = 1;
f1 = -a*x1^2 + x2 + u2*u3;
f2 = -x2 + b*x3 - u1*u3;
f3 = -c*x3^2 + exp(-u1);
F = [f1; f2; f3];

== matlab function control_mimo_simulink/PTO EQUILIBRIO MIMO NO LINEAL/Subsystem/MATLAB Function ==
  data: x input; u input; F output
function F = fcn(x,u)
x1 = x(1);
x2 = x(2);
x3 = x(3);
u1 = u(1);
u2 = u(2);
u3 = u(3);
a = 1;
b = 1;
c = 1;
f1 = -a*x1^2 + x2 + u2*u3;
f2 = -x2 + b*x3 - u1*u3;
f3 = -c*x3^2 + exp(-u1);
F = [f1; f2; f3];

== matlab function control_mimo_simulink/SEGUIMIENTO NO LINEAL/Subsystem/MATLAB Function ==
  data: x input; u input; F output
function F = fcn(x,u)
x1 = x(1);
x2 = x(2);
x3 = x(3);
u1 = u(1);
u2 = u(2);
u3 = u(3);
a = 1;
b = 1;
c = 1;
f1 = -a*x1^2 + x2 + u2*u3;
f2 = -x2 + b*x3 - u1*u3;
f3 = -c*x3^2 + exp(-u1);
F = [f1; f2; f3];

== matlab function control_mimo_simulink/SEGUIMIENTO NO LINEAL1/Subsystem/MATLAB Function ==
  data: x input; u input; F output
function F = fcn(x,u)
x1 = x(1);
x2 = x(2);
x3 = x(3);
u1 = u(1);
u2 = u(2);
u3 = u(3);
a = 1;
b = 1;
c = 1;
f1 = -a*x1^2 + x2 + u2*u3;
f2 = -x2 + b*x3 - u1*u3;
f3 = -c*x3^2 + exp(-u1);
F = [f1; f2; f3];

== matlab function control_mimo_simulink/SEGUIMIENTO NO LINEAL1/Subsystem2/MATLAB Function ==
  data: x input; u input; F output
function F = fcn(x,u)
x1 = x(1);
x2 = x(2);
x3 = x(3);
u1 = u(1);
u2 = u(2);
u3 = u(3);
a = 1;
b = 1;
c = 1;
f1 = -a*x1^2 + x2 + u2*u3;
f2 = -x2 + b*x3 - u1*u3;
f3 = -c*x3^2 + exp(-u1);
F = [f1; f2; f3];

== matlab function control_mimo_simulink/SEGUIMIENTO NO LINEAL1/Subsystem4/MATLAB Function ==
  data: x input; u input; F output
function F = fcn(x,u)
x1 = x(1);
x2 = x(2);
x3 = x(3);
u1 = u(1);
u2 = u(2);
u3 = u(3);
a = 1;
b = 1;
c = 1;
f1 = -a*x1^2 + x2 + u2*u3;
f2 = -x2 + b*x3 - u1*u3;
f3 = -c*x3^2 + exp(-u1);
F = [f1; f2; f3];
